simulink model "untitled"  (R2015a)
settings: Solver=FixedStepDiscrete  SolverMode=SingleTasking  StartTime=0.0  StopTime=100  FixedStep=1e-3  RelTol=1e-3
libraries: mbed_lib x7
settings Model: Creator=svenl  LastModifiedBy=svenl
settings OptimizationCC: OptimizeModelRefInitCode=on  LifeSpan=1
settings HardwareCC: ProdLargestAtomicInteger=Long  ProdLargestAtomicFloat=Double  ProdEndianess=LittleEndian  ProdHWDeviceType=ARM Compatible->ARM Cortex
settings RTWCC: SystemTargetFile=mbed.tlc  TemplateMakefile=mbed.tmf  Description=Mbed Target (Embedded Target)  TargetLang=C++
settings CodeAppCC: IgnoreCustomStorageClasses=off
settings STFCustomTargetCC: CombineOutputUpdateFcns=on  SupportContinuousTime=off  SupportVariableSizeSignals=off  SystemTargetFile=mbed.tlc
settings ERTTargetCC: SupportContinuousTime=off  SupportVariableSizeSignals=off  ERTCustomFileTemplate=mbed_file_process.tlc

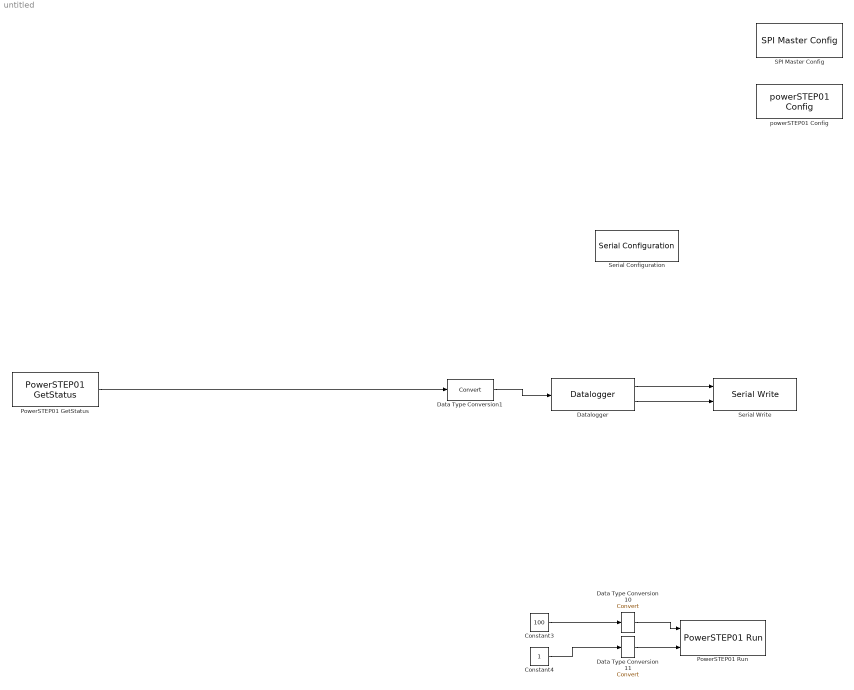
== system untitled ==
  Constant3 : Constant  Value=100
  Constant4 : Constant
  Data Type Conversion1 : DataTypeConversion
  Data Type Conversion10 : DataTypeConversion
  Data Type Conversion11 : DataTypeConversion
  Datalogger : mbed_lib/Utilities/Datalogger  TypeInputPorts={ 'double' 1 }  TypeOfInputs={'1*double' }  BufferSize=1000  errEn=off  SampleTime=-1
  PowerSTEP01 GetStatus : mbed_lib/SPI/PowerSTEP01 GetStatus  SPINr=1  NumMotors=1  SSELPort=B  SSELPin=6  SampleTime=1
  PowerSTEP01 Run : mbed_lib/SPI/PowerSTEP01 Run  SPINr=1  NumMotors=1  SSELPort=B  SSELPin=6  SampleTime=1
  SPI Master Config : mbed_lib/SPI/SPI Master Config  Priority=0  SpiPort=1  SpiFreq=100000  MosiPort=A  MosiPin=7  MisoPort=A  MisoPin=6  SclkPort=A  SclkPin=5
  Serial Configuration : mbed_lib/Serial/Serial Configuration  SerialPort=1  TXPort=A  TXPin=2  RXPort=A  RXPin=3  BaudRate=115200
  Serial Write : mbed_lib/Serial/Serial Write  SerialPort=1  numData=on  SampleTime=-1
  "powerSTEP01 Config " : mbed_lib/SPI/powerSTEP01 Config   Priority=0  SPINr=1  SSELPort=B  SSELPin=6  ResetPort=A  ResetPin=10  ACC=50  DEC=50  MaxSpeed=1000  MinSpeed=0  FullStepSpeed=200  Overcurrent=300  StepMode=STEP_MODE_1_16  CurrentVoltageModeSEL=on  Holdtorque=2  Runtorque=2  ACCtorque=2  DECtorque=2  Motor2SEL=on  ACC_1=100  DEC_1=50  MaxSpeed_1=300  MinSpeed_1=0  FullStepSpeed_1=300  Overcurrent_1=300  StepMode_1=STEP_MODE_1_64  CurrentVoltageModeSEL_1=on  Holdtorque_1=20  Runtorque_1=50  ACCtorque_1=120  DECtorque_1=120  Motor3SEL=off  ACC_2=0  DEC_2=0  MaxSpeed_2=0  MinSpeed_2=0  FullStepSpeed_2=0  Overcurrent_2=0  StepMode_2=STEP_MODE_FULL  CurrentVoltageModeSEL_2=on  Holdtorque_2=0  Runtorque_2=0  ACCtorque_2=0  DECtorque_2=0
  wires:
  Datalogger/1 -> Serial Write/1
  Datalogger/2 -> Serial Write/2
  Data Type Conversion1/1 -> Datalogger/1
  PowerSTEP01 GetStatus/1 -> Data Type Conversion1/1
  Constant4/1 -> Data Type Conversion11/1
  Constant3/1 -> Data Type Conversion10/1
  Data Type Conversion10/1 -> PowerSTEP01 Run/1
  Data Type Conversion11/1 -> PowerSTEP01 Run/2
